simulink model "verify_Hot_Water_Consumption_EN13203_mdl"  (R2016b)
settings: Solver=ode45  StartTime=0.0  StopTime=24*3600  MaxStep=900  RelTol=1e-3  EnableMultiTasking=on
libraries: carnot x4
settings Model: DEBUGGLOBALLEVEL=DEBUGLEVEL  DEBUGMAXTOTALWARNINGS=0  DEBUGMAXCONSECUTIVEWARNINGS=0  DEBUGWRITETOFILE=0  DEBUGFILENAME='error.txt'  Creator=drhf  LastModifiedBy=drhf
settings DataIOCC: SaveFormat=Array  SignalLoggingSaveFormat=ModelDataLogs
settings OptimizationCC: ExpressionDepthLimit=2147483647  LifeSpan=inf
settings DebuggingCC: UnderspecifiedInitializationDetection=Classic  MergeDetectMultiDrivingBlocksExec=none  SolverPrmCheckMsg=warning  FcnCallInpInsideContextMsg=warning  StateNameClashWarn=warning  SFUnexpectedBacktrackingDiag=warning  SFNoUnconditionalDefaultTransitionDiag=warning  SFExecutionAtInitializationDiag=none
settings HardwareCC: ProdBitPerPointer=32  ProdBitPerSizeT=32  ProdBitPerPtrDiffT=32  ProdLargestAtomicFloat=None  ProdIntDivRoundTo=Undefined  ProdEndianess=Unspecified  ProdWordSize=32  ProdHWDeviceType=32-bit Generic
settings ModelReferenceCC: PropagateSignalLabelsOutOfModel=off
settings GRTTargetCC: TargetLangStandard=C89/C90 (ANSI)  GeneratePreprocessorConditionals=Disable all  CombineOutputUpdateFcns=off  GRTInterface=on
settings ConfigComp: CovMetricSettings=dw  CovHtmlReporting=on  CovSaveCumulativeToWorkspaceVar=on  CovSaveSingleToWorkspaceVar=on  CovExternalEMLEnable=off

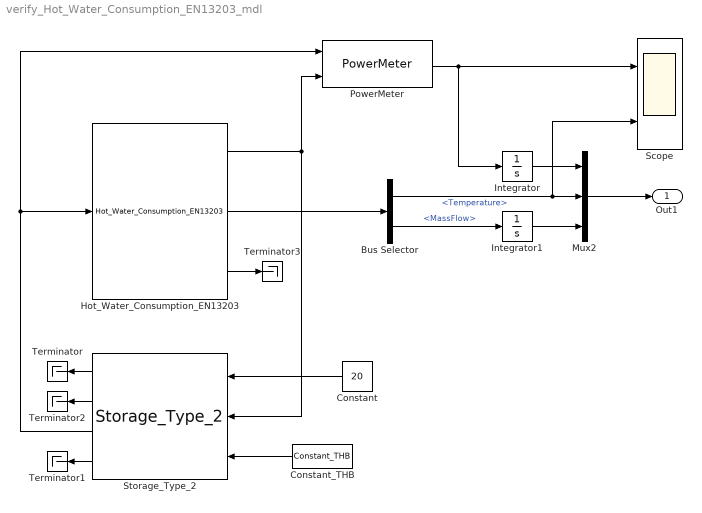
== system verify_Hot_Water_Consumption_EN13203_mdl ==
  Bus Selector : BusSelector  OutputSignals=Temperature,MassFlow
  Constant : Constant  Value=20
  Constant_THB : carnot/Source/Simple/Constant_THB  t=60  mdot=1000/3600  p=1e5  mID=No Pressure Drop  fluid=Water  mix=0  mix2=0  mix3=0  dia=0.02  hgt=0
  Hot_Water_Consumption_EN13203 : carnot/Load/Hot_Water_Tapping/Applications/Hot_Water_Consumption_EN13203  SystemSampleTime=-1
  Integrator : Integrator
  Integrator1 : Integrator
  Mux2 : Mux  Inputs=3
  PowerMeter : carnot/Control/PowerMeter
  Scope : Scope  NumInputPorts=2
  Storage_Type_2 : carnot/Storage/Thermal/Storage_Type_2  uloss=1  ubot=1  utop=1  cond=1  volume=0.3  dia=0.5  pos=standing cylinder  h_in_chg=0.5  h_out_chg=0.1  ua0=200  uam=0.2  uat=0.5  dplin_chg=100  dpqua_chg=100  h_in=0  h_out=1  pipedia=0.03  t0=60  nodes=10  mpoints=10
  Terminator{,1..3} (4 alike) : Terminator
  Out1 : Outport
  wires:
  Mux2/1 -> Out1/1
  Storage_Type_2/3 -> PowerMeter/1, Hot_Water_Consumption_EN13203/1
  Hot_Water_Consumption_EN13203/1 -> Storage_Type_2/2, PowerMeter/2
  Storage_Type_2/1 -> Terminator/1
  Storage_Type_2/4 -> Terminator1/1
  Constant_THB/1 -> Storage_Type_2/3
  Constant/1 -> Storage_Type_2/1
  Storage_Type_2/2 -> Terminator2/1
  Hot_Water_Consumption_EN13203/3 -> Terminator3/1
  Hot_Water_Consumption_EN13203/2 -> Bus Selector/1
  Bus Selector/1 -> Scope/2, Mux2/2  "<Temperature>"
  Bus Selector/2 -> Integrator1/1  "<MassFlow>"
  PowerMeter/1 -> Integrator/1, Scope/1
  Integrator/1 -> Mux2/1
  Integrator1/1 -> Mux2/3
